simulink model "PID_Soplado_PE"  (R2020b)
settings: Solver=VariableStepAuto  StartTime=0.0  StopTime=10.0  RelTol=1e-3
settings Model: Creator=bou  LastModifiedBy=bou

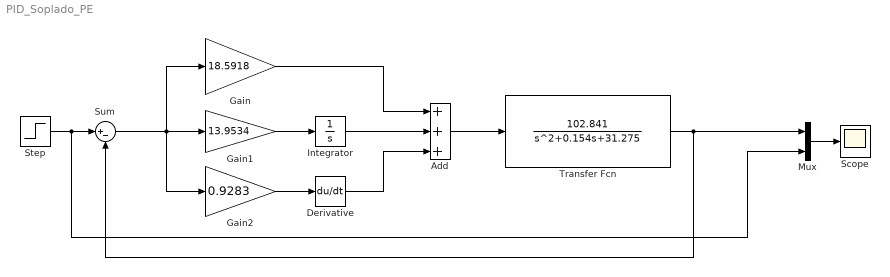
== system PID_Soplado_PE ==
  Add : Sum  Inputs=+++
  Derivative : Derivative
  Gain : Gain  Gain=18.5918
  Gain1 : Gain  Gain=13.9534
  Gain2 : Gain  Gain=0.9283
  Integrator : Integrator
  Mux : Mux  Inputs=2
  Scope : Scope
  Step : Step  After=3.3  SampleTime=0
  Sum : Sum  Inputs=|+-
  Transfer Fcn : TransferFcn  Numerator=[102.841]  Denominator=[1 0.154 31.275]
  wires:
  Integrator/1 -> Add/2
  Derivative/1 -> Add/3
  Gain/1 -> Add/1
  Gain1/1 -> Integrator/1
  Gain2/1 -> Derivative/1
  Sum/1 -> Gain/1, Gain1/1, Gain2/1
  Add/1 -> Transfer Fcn/1
  Transfer Fcn/1 -> Mux/1, Sum/2
  Step/1 -> Mux/2, Sum/1
  Mux/1 -> Scope/1
